simulink subsystem "bh_COMP_sys_Lagrange"  (R2022b)
settings: Solver=VariableStepAuto  StartTime=0.0  StopTime=10.0  RelTol=1e-3
undefined symbols (not defined in the file or in its folder): IC_T, params_T
libraries: simulink x1, simulink_extras x1
settings Model: Creator=bhorton  LastModifiedBy=bhorton
settings DebuggingCC: UnconnectedInputMsg=warning  UnconnectedOutputMsg=warning  UnconnectedLineMsg=warning
settings ModelReferenceCC: EnableRefExpFcnMdlSchedulingChecks=on
settings RTWCC: DLArmComputeVersion=19.05

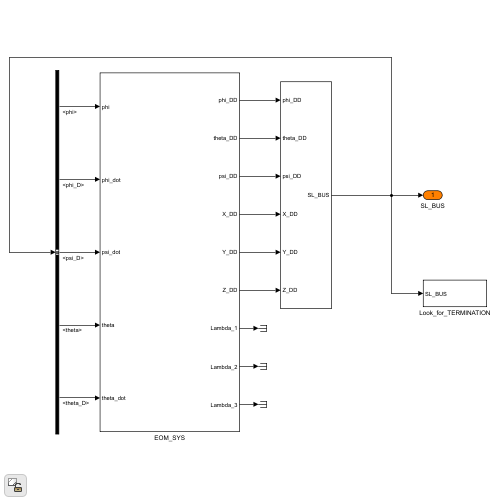
[thumbnail: Simulink's stored preview of the top-level diagram]
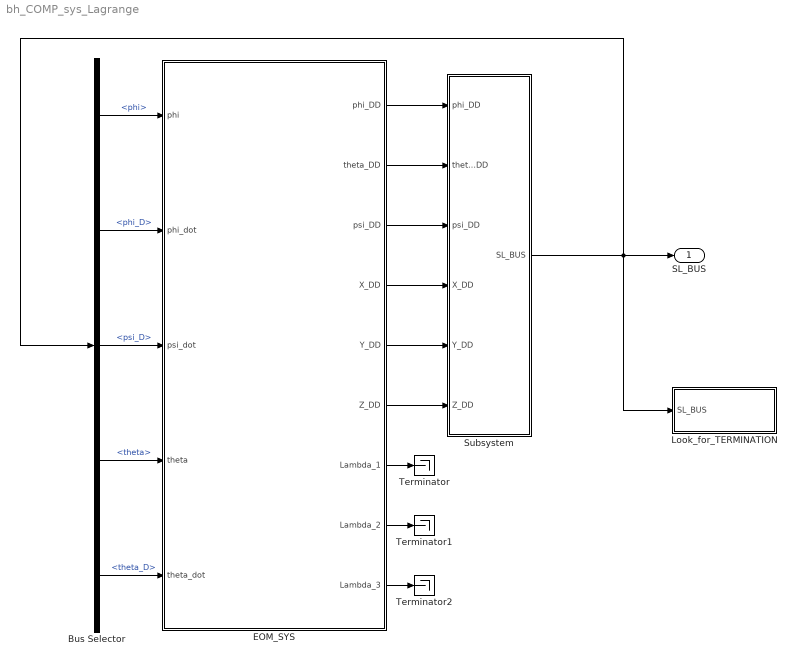
== system bh_COMP_sys_Lagrange ==
  Bus Selector : BusSelector  OutputSignals=phi,phi_D,psi_D,theta,theta_D
  EOM_SYS : Subsystem
  Look_for_TERMINATION : Subsystem
  Subsystem : Subsystem
  Terminator : Terminator
  Terminator1 : Terminator
  Terminator2 : Terminator
  SL_BUS : Outport
  wires:
  EOM_SYS/6(Z_DD) -> Subsystem/6(Z_DD)
  EOM_SYS/5(Y_DD) -> Subsystem/5(Y_DD)
  EOM_SYS/4(X_DD) -> Subsystem/4(X_DD)
  EOM_SYS/3(psi_DD) -> Subsystem/3(psi_DD)
  EOM_SYS/2(theta_DD) -> Subsystem/2(theta_DD)
  EOM_SYS/1(phi_DD) -> Subsystem/1(phi_DD)
  Bus Selector/3 -> EOM_SYS/3(psi_dot)  "<psi_D>"
  Bus Selector/2 -> EOM_SYS/2(phi_dot)  "<phi_D>"
  Bus Selector/1 -> EOM_SYS/1(phi)  "<phi>"
  Bus Selector/4 -> EOM_SYS/4(theta)  "<theta>"
  Bus Selector/5 -> EOM_SYS/5(theta_dot)  "<theta_D>"
  Subsystem/1(SL_BUS) -> Bus Selector/1, SL_BUS/1, Look_for_TERMINATION/1(SL_BUS)
  EOM_SYS/7(Lambda_1) -> Terminator/1
  EOM_SYS/8(Lambda_2) -> Terminator1/1
  EOM_SYS/9(Lambda_3) -> Terminator2/1

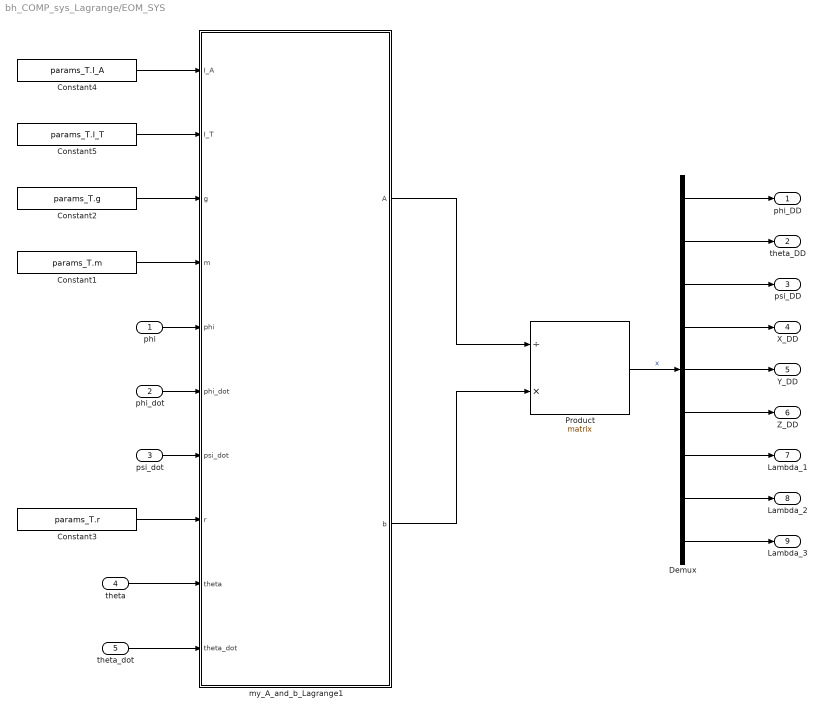
== system bh_COMP_sys_Lagrange/EOM_SYS ==
  phi : Inport
  phi_dot : Inport  Port=2
  psi_dot : Inport  Port=3
  theta : Inport  Port=4
  theta_dot : Inport  Port=5
  Constant1 : Constant  Value=params_T.m
  Constant2 : Constant  Value=params_T.g
  Constant3 : Constant  Value=params_T.r
  Constant4 : Constant  Value=params_T.I_A
  Constant5 : Constant  Value=params_T.I_T
  Demux : Demux  Outputs=9
  Product : Product  Inputs=/*  Multiplication=Matrix(*)
  my_A_and_b_Lagrange1 : MATLAB Function  TreatAsAtomicUnit=on
  phi_DD : Outport
  theta_DD : Outport  Port=2
  psi_DD : Outport  Port=3
  X_DD : Outport  Port=4
  Y_DD : Outport  Port=5
  Z_DD : Outport  Port=6
  Lambda_1 : Outport  Port=7
  Lambda_2 : Outport  Port=8
  Lambda_3 : Outport  Port=9
  wires:
  Constant5/1 -> my_A_and_b_Lagrange1/2(I_T)
  Constant4/1 -> my_A_and_b_Lagrange1/1(I_A)
  Constant2/1 -> my_A_and_b_Lagrange1/3(g)
  Constant1/1 -> my_A_and_b_Lagrange1/4(m)
  theta/1 -> my_A_and_b_Lagrange1/9(theta)
  theta_dot/1 -> my_A_and_b_Lagrange1/10(theta_dot)
  psi_dot/1 -> my_A_and_b_Lagrange1/7(psi_dot)
  phi_dot/1 -> my_A_and_b_Lagrange1/6(phi_dot)
  Demux/9 -> Lambda_3/1
  Demux/8 -> Lambda_2/1
  Demux/7 -> Lambda_1/1
  Demux/6 -> Z_DD/1
  Demux/5 -> Y_DD/1
  Demux/4 -> X_DD/1
  Demux/3 -> psi_DD/1
  Demux/2 -> theta_DD/1
  phi/1 -> my_A_and_b_Lagrange1/5(phi)
  Constant3/1 -> my_A_and_b_Lagrange1/8(r)
  my_A_and_b_Lagrange1/2(b) -> Product/2
  my_A_and_b_Lagrange1/1(A) -> Product/1
  Demux/1 -> phi_DD/1
  Product/1 -> Demux/1  "x"

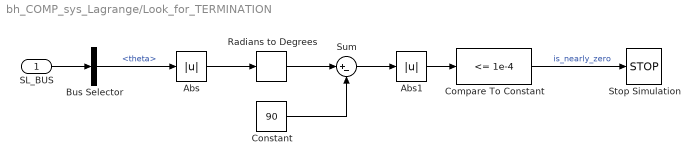
== system bh_COMP_sys_Lagrange/Look_for_TERMINATION ==
  SL_BUS : Inport
  Abs : Abs  SaturateOnIntegerOverflow=off
  Abs1 : Abs  SaturateOnIntegerOverflow=off
  Bus Selector : BusSelector  OutputSignals=theta
  Compare To Constant : simulink/Logic and Bit Operations/Compare To Constant  relop=<=  const=1e-4  OutDataTypeStr=boolean
  Constant : Constant  Value=90
  Radians to Degrees : simulink_extras/Transformations/Radians to Degrees
  Stop Simulation : Stop
  Sum : Sum  Inputs=|+-
  wires:
  Compare To Constant/1 -> Stop Simulation/1  "is_nearly_zero"
  Abs1/1 -> Compare To Constant/1
  Sum/1 -> Abs1/1
  Constant/1 -> Sum/2
  Radians to Degrees/1 -> Sum/1
  Abs/1 -> Radians to Degrees/1
  Bus Selector/1 -> Abs/1  "<theta>"
  SL_BUS/1 -> Bus Selector/1

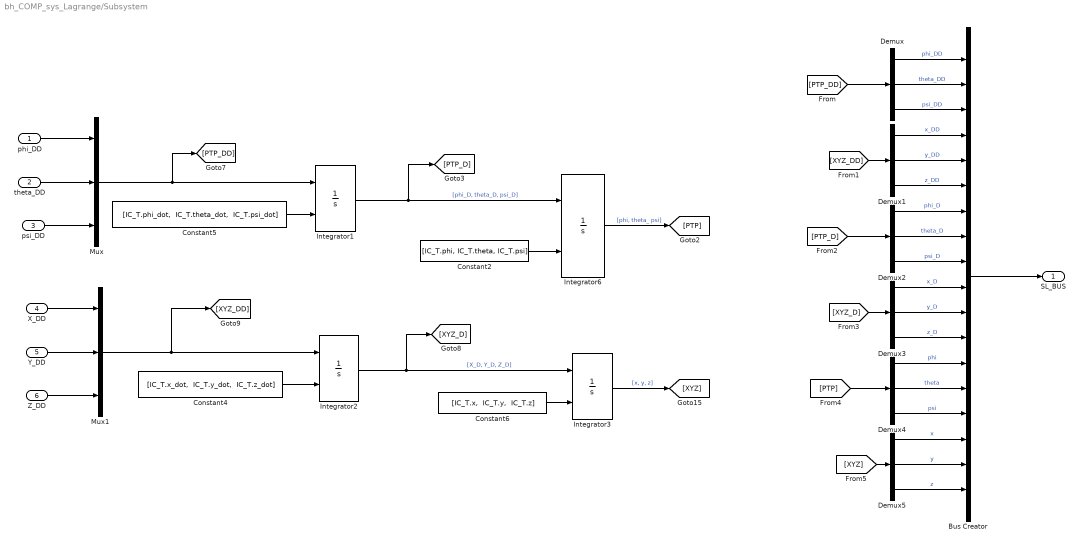
== system bh_COMP_sys_Lagrange/Subsystem ==
  phi_DD : Inport
  theta_DD : Inport  Port=2
  psi_DD : Inport  Port=3
  X_DD : Inport  Port=4
  Y_DD : Inport  Port=5
  Z_DD : Inport  Port=6
  Bus Creator : BusCreator  Inputs=18
  Constant2 : Constant  Value="[IC_T.phi,  IC_T.theta,  IC_T.psi]"
  Constant4 : Constant  Value="[IC_T.x_dot,  IC_T.y_dot,  IC_T.z_dot]"
  Constant5 : Constant  Value="[IC_T.phi_dot,  IC_T.theta_dot,  IC_T.psi_dot]"
  Constant6 : Constant  Value="[IC_T.x,  IC_T.y,  IC_T.z]"
  Demux{,1..5} (6 alike) : Demux  Outputs=3
  Integrator1 : Integrator  InitialConditionSource=external
  Integrator2 : Integrator  InitialConditionSource=external
  Integrator3 : Integrator  InitialConditionSource=external
  Integrator6 : Integrator  InitialConditionSource=external  WrapState=on  WrappedStateUpperValue=2*pi  WrappedStateLowerValue=0  AbsoluteTolerance=1e-8
  Mux : Mux  Inputs=3
  Mux1 : Mux  Inputs=3
  SL_BUS : Outport
  wires:
  [XYZ] -> Demux5/1
  [PTP] -> Demux4/1
  [XYZ_D] -> Demux3/1
  [PTP_D] -> Demux2/1
  [XYZ_DD] -> Demux1/1
  [PTP_DD] -> Demux/1
  Demux4/3 -> Bus Creator/15  "psi"
  Demux5/1 -> Bus Creator/16  "x"
  Demux5/3 -> Bus Creator/18  "z"
  Demux4/1 -> Bus Creator/13  "phi"
  Demux4/2 -> Bus Creator/14  "theta"
  Demux5/2 -> Bus Creator/17  "y"
  Demux2/3 -> Bus Creator/9  "psi_D"
  Demux3/2 -> Bus Creator/11  "y_D"
  Demux3/1 -> Bus Creator/10  "x_D"
  Demux3/3 -> Bus Creator/12  "z_D"
  Demux2/1 -> Bus Creator/7  "phi_D"
  Demux2/2 -> Bus Creator/8  "theta_D"
  Demux1/3 -> Bus Creator/6  "z_DD"
  Demux1/2 -> Bus Creator/5  "y_DD"
  Demux1/1 -> Bus Creator/4  "x_DD"
  Demux/3 -> Bus Creator/3  "psi_DD"
  Demux/1 -> Bus Creator/1  "phi_DD"
  Demux/2 -> Bus Creator/2  "theta_DD"
  Bus Creator/1 -> SL_BUS/1
  Mux1/1 -> Integrator2/1, [XYZ_DD]
  Constant4/1 -> Integrator2/2
  Integrator3/1 -> [XYZ]  "[x, y, z]"
  X_DD/1 -> Mux1/1
  Y_DD/1 -> Mux1/2
  Z_DD/1 -> Mux1/3
  Mux/1 -> Integrator1/1, [PTP_DD]
  phi_DD/1 -> Mux/1
  theta_DD/1 -> Mux/2
  psi_DD/1 -> Mux/3
  Constant5/1 -> Integrator1/2
  Constant2/1 -> Integrator6/2
  Integrator6/1 -> [PTP]  "[phi, theta_ psi]"
  Integrator1/1 -> [PTP_D], Integrator6/1  "[phi_D, theta_D, psi_D]"
  Integrator2/1 -> Integrator3/1, [XYZ_D]  "[X_D, Y_D, Z_D]"
  Constant6/1 -> Integrator3/2

== matlab function bh_COMP_sys_Lagrange/EOM_SYS/my_A_and_b_Lagrange1 ==
  data: I_A input; A output; I_T input; g input; m input; phi input; phi_dot input; psi_dot input; r input; theta input; theta_dot input; b output
function [A,b] = my_A_and_b_Lagrange(I_A,I_T,g,m,phi,phi_dot,psi_dot,r,theta,theta_dot)
%#codegen

%    This function was generated by the Symbolic Math Toolbox version 9.2.
%    27-Oct-2022 13:34:55

A = reshape([I_A-I_A.*cos(theta).^2+I_T.*cos(theta).^2,0.0,-I_A.*sin(theta),0.0,0.0,0.0,r.*sin(phi).*sin(theta),-r.*cos(phi).*sin(theta),0.0,0.0,I_T,0.0,0.0,0.0,0.0,-r.*cos(phi).*cos(theta),-r.*cos(theta).*sin(phi),r.*sin(theta),-I_A.*sin(theta),0.0,I_A,0.0,0.0,0.0,-r.*sin(phi),r.*cos(phi),0.0,0.0,0.0,0.0,m,0.0,0.0,1.0,0.0,0.0,0.0,0.0,0.0,0.0,m,0.0,0.0,1.0,0.0,0.0,0.0,0.0,0.0,0.0,m,0.0,0.0,1.0,r.*sin(phi).*sin(theta),-r.*cos(phi).*cos(theta),-r.*sin(phi),1.0,0.0,0.0,0.0,0.0,0.0,-r.*cos(phi).*sin(theta),-r.*cos(theta).*sin(phi),r.*cos(phi),0.0,1.0,0.0,0.0,0.0,0.0,0.0,r.*sin(theta),0.0,0.0,0.0,1.0,0.0,0.0,0.0],[9,9]);
if nargout > 1
    b = [I_A.*psi_dot.*theta_dot.*cos(theta)-I_A.*phi_dot.*theta_dot.*sin(theta.*2.0)+I_T.*phi_dot.*theta_dot.*sin(theta.*2.0);(I_A.*phi_dot.^2.*sin(theta.*2.0))./2.0-(I_T.*phi_dot.^2.*sin(theta.*2.0))./2.0-I_A.*phi_dot.*psi_dot.*cos(theta);I_A.*phi_dot.*theta_dot.*cos(theta);0.0;0.0;-g.*m;-r.*(-phi_dot.*psi_dot.*cos(phi)+phi_dot.^2.*cos(phi).*sin(theta)+theta_dot.^2.*cos(phi).*sin(theta)+phi_dot.*theta_dot.*cos(theta).*sin(phi).*2.0);r.*(phi_dot.*psi_dot.*sin(phi)-phi_dot.^2.*sin(phi).*sin(theta)-theta_dot.^2.*sin(phi).*sin(theta)+phi_dot.*theta_dot.*cos(phi).*cos(theta).*2.0);-r.*theta_dot.^2.*cos(theta)];
end
